simulink model "final_system"  (R2022b)
settings: Solver=VariableStepAuto  StartTime=0.0  StopTime=20  RelTol=1e-3
values from neighbouring files (symbols this model uses):
  omega0 = 904    [Exam_TB1_Control.m]    (also in final_fusion.m = 1)
settings Model: Creator=zd012  LastModifiedBy=zd012
settings DebuggingCC: UnconnectedInputMsg=warning  UnconnectedOutputMsg=warning  UnconnectedLineMsg=warning
settings ModelReferenceCC: EnableRefExpFcnMdlSchedulingChecks=on
settings RTWCC: DLArmComputeVersion=19.05

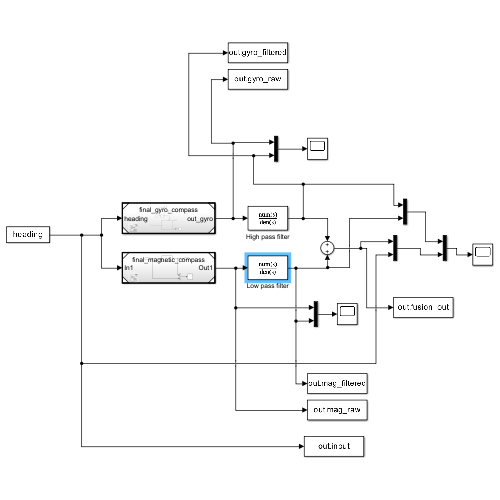
[thumbnail: Simulink's stored preview of the top-level diagram]
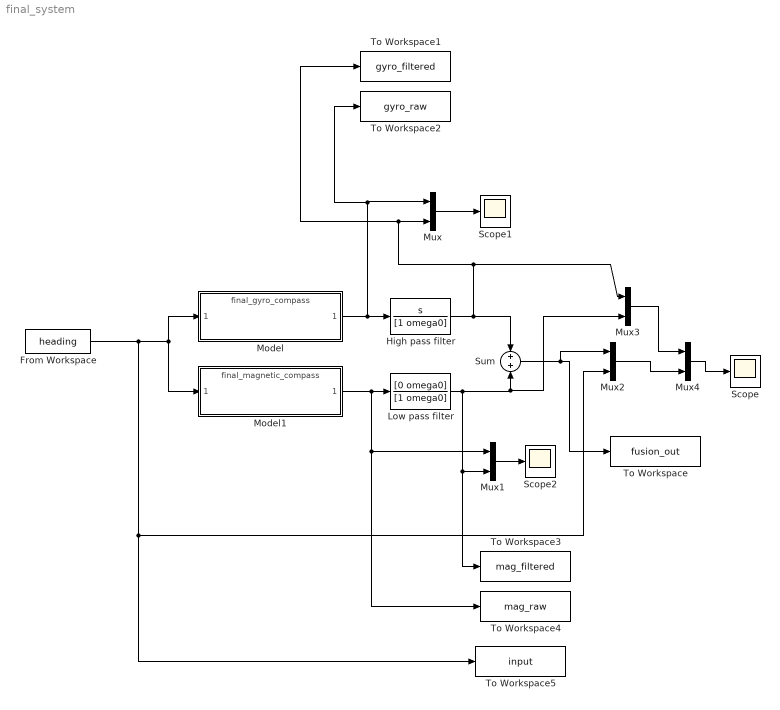
== system final_system ==
  From Workspace : FromWorkspace  VariableName=heading
  High pass filter : TransferFcn  Numerator=[1 0]  Denominator=[1 omega0]
  Low pass filter : TransferFcn  Numerator=[0 omega0]  Denominator=[1 omega0]
  Model : ModelReference  ModelNameDialog=final_gyro_compass  SimulationMode=Normal  ModelReferenceVersion=1.3
  Model1 : ModelReference  ModelNameDialog=final_magnetic_compass  SimulationMode=Normal  ModelReferenceVersion=1.8
  Mux{,1..4} (5 alike) : Mux  Inputs=2
  Scope : Scope
  Scope1 : Scope
  Scope2 : Scope
  Sum : Sum  Inputs=+|+
  To Workspace : ToWorkspace  VariableName=fusion_out  SampleTime=-1
      settings: Save2DSignal=2-D array (concatenate along first dimension)
  To Workspace1 : ToWorkspace  VariableName=gyro_filtered  SampleTime=-1
      settings: Save2DSignal=2-D array (concatenate along first dimension)
  To Workspace2 : ToWorkspace  VariableName=gyro_raw  SampleTime=-1
      settings: Save2DSignal=2-D array (concatenate along first dimension)
  To Workspace3 : ToWorkspace  VariableName=mag_filtered  SampleTime=-1
      settings: Save2DSignal=2-D array (concatenate along first dimension)
  To Workspace4 : ToWorkspace  VariableName=mag_raw  SampleTime=-1
      settings: Save2DSignal=2-D array (concatenate along first dimension)
  To Workspace5 : ToWorkspace  VariableName=input  SampleTime=-1
      settings: Save2DSignal=2-D array (concatenate along first dimension)
  wires:
  From Workspace/1 -> To Workspace5/1, Mux2/2, Model1/1, Model/1
  Model/1 -> To Workspace2/1, Mux/1, High pass filter/1
  High pass filter/1 -> To Workspace1/1, Mux/2, Mux3/1, Sum/1
  Mux/1 -> Scope1/1
  Model1/1 -> To Workspace4/1, Mux1/1, Low pass filter/1
  Mux1/1 -> Scope2/1
  Low pass filter/1 -> To Workspace3/1, Mux1/2, Mux3/2, Sum/2
  Sum/1 -> To Workspace/1, Mux2/1
  Mux4/1 -> Scope/1
  Mux2/1 -> Mux4/2
  Mux3/1 -> Mux4/1
